simulink model "GenData"  (R2014a)
settings: Solver=FixedStepDiscrete  StartTime=0.0  StopTime=20  FixedStep=SampleTime  RelTol=1e-3
values from neighbouring files (symbols this model uses):
  SampleTime = evalin('base','SampleTime')    [FIDF_Design.m]    (also in FIDF_Designing.m; FIDF_Framework.m; default_settings.m = 0.01; set_global_callback.m = 0.01)
undefined symbols (not defined in the file or in its folder): mean_noise, mean_outlier, var_noise, var_outlier
libraries: simulink x2
settings Model: Creator=georg  LastModifiedBy=georg

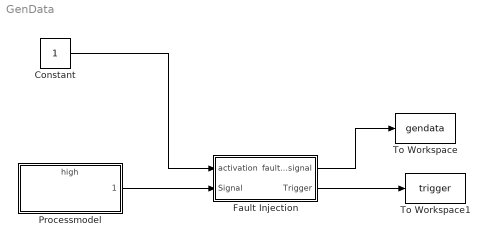
== system GenData ==
  Constant : Constant
  Fault Injection : Subsystem
  Processmodel : ModelReference  ModelNameDialog=high.slx  SimulationMode=Normal  ModelReferenceVersion=1.14  CopyOfModelName=high.slx  DefaultDataLogging=on
  To Workspace : ToWorkspace  VariableName=gendata  SampleTime=-1
  To Workspace1 : ToWorkspace  VariableName=trigger  SampleTime=-1
  wires:
  Processmodel/1 -> Fault Injection/2(Signal)
  Fault Injection/1(faulty_signal) -> To Workspace/1
  Constant/1 -> Fault Injection/1(activation)
  Fault Injection/2(Trigger) -> To Workspace1/1

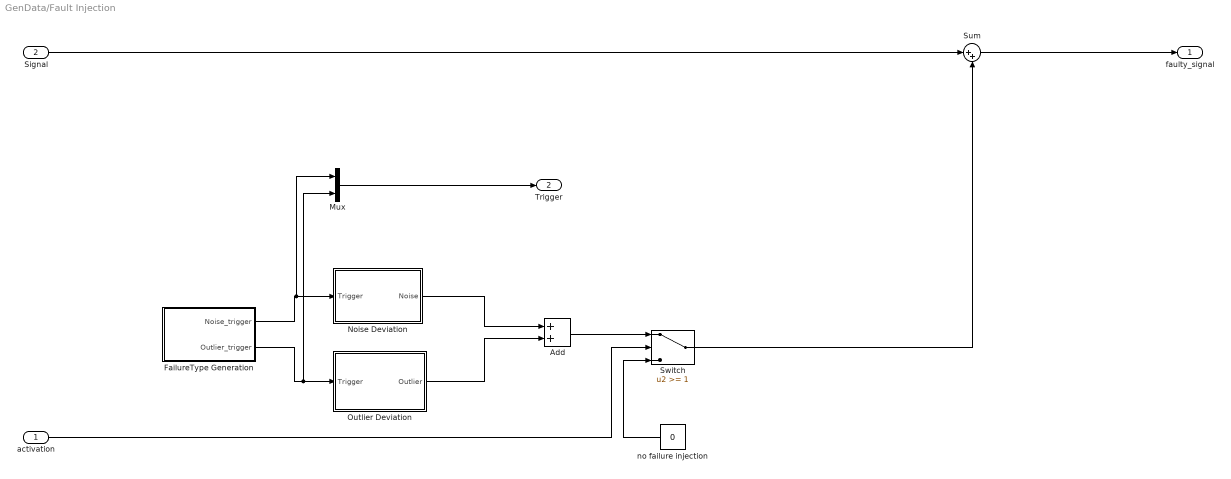
== system GenData/Fault Injection ==
  activation : Inport
  Signal : Inport  Port=2
  Add : Sum
  FailureType Generation : Subsystem
  Mux : Mux  Inputs=2
  Noise Deviation : Subsystem
  Outlier Deviation : Subsystem
  Sum : Sum  Inputs=|++
  Switch : Switch  Threshold=1
  no failure injection : Constant  Value=0
  faulty_signal : Outport
  Trigger : Outport  Port=2
  wires:
  Noise Deviation/1(Noise) -> Add/1
  Outlier Deviation/1(Outlier) -> Add/2
  no failure injection/1 -> Switch/3
  Add/1 -> Switch/1
  Switch/1 -> Sum/2
  activation/1 -> Switch/2
  FailureType Generation/1(Noise_trigger) -> Mux/1, Noise Deviation/1(Trigger)
  FailureType Generation/2(Outlier_trigger) -> Mux/2, Outlier Deviation/1(Trigger)
  Sum/1 -> faulty_signal/1
  Signal/1 -> Sum/1
  Mux/1 -> Trigger/1

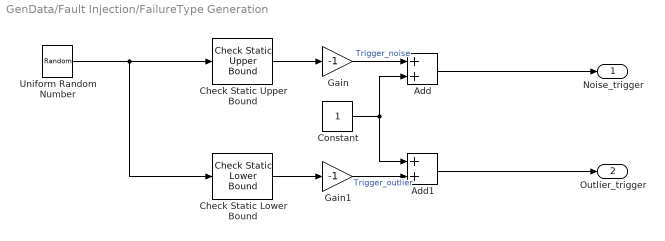
== system GenData/Fault Injection/FailureType Generation ==
  Add : Sum
  Add1 : Sum
  Check Static Lower Bound : simulink/Model Verification/Check Static  Lower Bound  Description=prob_outlier <= u  min=prob_outlier  min_included=on  enabled=off  stopWhenAssertionFail=off  export=on  icon=graphic
  Check Static Upper Bound : simulink/Model Verification/Check Static  Upper Bound  Description=u <= prob_noise  max=prob_noise  max_included=on  enabled=off  stopWhenAssertionFail=off  export=on  icon=graphic
  Constant : Constant
  Gain : Gain  Gain=-1
  Gain1 : Gain  Gain=-1
  Uniform Random Number : UniformRandomNumber  Seed=1  SampleTime=SampleTime
  Noise_trigger : Outport
  Outlier_trigger : Outport  Port=2
  wires:
  Uniform Random Number/1 -> Check Static Lower Bound/1, Check Static Upper Bound/1
  Check Static Upper Bound/1 -> Gain/1
  Check Static Lower Bound/1 -> Gain1/1
  Gain1/1 -> Add1/2  "Trigger_outlier"
  Gain/1 -> Add/1  "Trigger_noise"
  Add1/1 -> Outlier_trigger/1
  Constant/1 -> Add1/1, Add/2
  Add/1 -> Noise_trigger/1

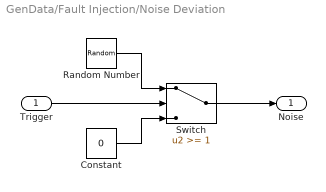
== system GenData/Fault Injection/Noise Deviation ==
  Trigger : Inport
  Constant : Constant  Value=0  SampleTime=SampleTime
  Random Number : RandomNumber  Mean=mean_noise  Variance=var_noise  SampleTime=SampleTime
  Switch : Switch  Threshold=1
  Noise : Outport
  wires:
  Constant/1 -> Switch/3
  Trigger/1 -> Switch/2
  Switch/1 -> Noise/1
  Random Number/1 -> Switch/1

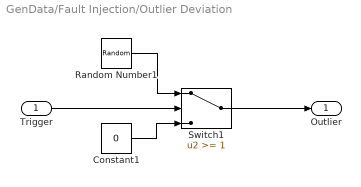
== system GenData/Fault Injection/Outlier Deviation ==
  Trigger : Inport
  Constant1 : Constant  Value=0
  Random Number1 : RandomNumber  Mean=mean_outlier  Variance=var_outlier  SampleTime=SampleTime
  Switch1 : Switch  Threshold=1
  Outlier : Outport
  wires:
  Constant1/1 -> Switch1/3
  Random Number1/1 -> Switch1/1
  Trigger/1 -> Switch1/2
  Switch1/1 -> Outlier/1
